simulink model "CoPT_TrqDesCoord1"  (R2016b)
settings: configuration reference "CodeGenConfigSet" (kept outside this file)
values from neighbouring files (symbols this model uses):
  DCS_OVRDS_ENGPRT = fi(1,State_int32)    [init_CoPT_TrqDesCoord.m]    (also in init_CoPT_TrqDesCoord_SIL.m)
  DCSOVRDSENGPRT_SY = fi(1,State_int32)    [init_CoPT_TrqDesCoord.m]    (also in init_CoPT_TrqDesCoord_SIL.m)
  DFFTLPRT_OVRDS_TSCINC = fi(1,State_int32)    [init_CoPT_TrqDesCoord.m]    (also in init_CoPT_TrqDesCoord_SIL.m)
  DFFTLPRTOVRDSTSCINC_SY = fi(1,State_int32)    [init_CoPT_TrqDesCoord.m]    (also in init_CoPT_TrqDesCoord_SIL.m)
  PTPRT_OVRDS_SPDGOV = fi(1,State_int32)    [init_CoPT_TrqDesCoord.m]    (also in init_CoPT_TrqDesCoord_SIL.m)
  PTPRTOVRDSSPDGOV_SY = fi(0,State_int32)    [init_CoPT_TrqDesCoord.m]    (also in init_CoPT_TrqDesCoord_SIL.m)
libraries: simulink x6
settings Model: Creator=Wollf  LastModifiedBy=lenovo
settings ConfigSetRef: SourceLocation=Base Workspace

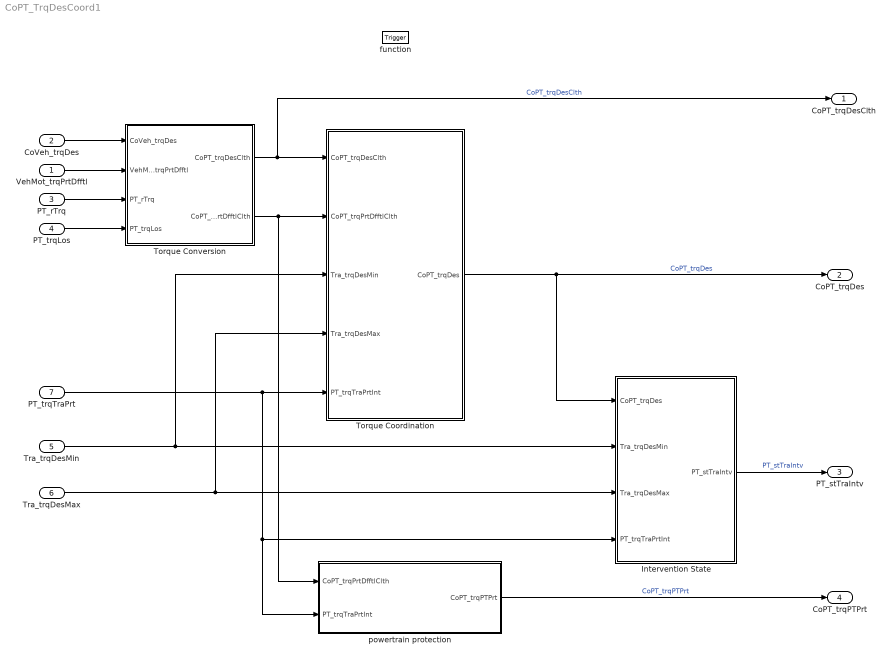
== system CoPT_TrqDesCoord1 ==
  VehMot_trqPrtDfftl : Inport  Tag=Nm  Description=Differential protection torque  OutMin=-3000  OutMax=3000  OutDataTypeStr=Trq_Nm
  CoVeh_trqDes : Inport  Tag=Nm  Description=Setpoint torque order to the drive train (gearbox output torque)  Port=2  OutMin=-3000  OutMax=3000  OutDataTypeStr=Trq_Nm
  PT_rTrq : Inport  Description=Powertrain torque ratio  Port=3  OutMin=-100  OutMax=100  OutDataTypeStr=TransRatio
  PT_trqLos : Inport  Tag=Nm  Description=Parameter for loss torque of the drive train  Port=4  OutMin=-3000  OutMax=3000  OutDataTypeStr=Trq_Nm
  Tra_trqDesMin : Inport  Tag=Nm  Description=Increment torque demand from gearbox  Port=5  OutMin=-3000  OutMax=3000  OutDataTypeStr=Trq_Nm
  Tra_trqDesMax : Inport  Tag=Nm  Description=Decrement torque demand from gearbox  Port=6  OutMin=-3000  OutMax=3000  OutDataTypeStr=Trq_Nm
  PT_trqTraPrt : Inport  Tag=Nm  Description=Maximum allowed inner torque  Port=7  OutMin=-3000  OutMax=3000  OutDataTypeStr=Trq_Nm
  function : TriggerPort  TriggerType=function-call  VariantControl=Variant
  Intervention State : Subsystem
  Torque Conversion : Subsystem
  Torque Coordination : Subsystem
  powertrain protection : Subsystem
  CoPT_trqDesClth : Outport  Tag=Nm  Description=Desired Clutch Torque  OutMin=-3000  OutMax=3000  OutDataTypeStr=Trq_Nm
  CoPT_trqDes : Outport  Tag=Nm  Description=Total torque order for torque actuator (clutch torque)  Port=2  OutMin=-3000  OutMax=3000  OutDataTypeStr=Trq_Nm
  PT_stTraIntv : Outport  Description=Status of torque access gearbox interventions  Port=3  OutMin=0  OutMax=255  OutDataTypeStr=State_uint8
  CoPT_trqPTPrt : Outport  Tag=Nm  Description=Drive train protection torque (clutch torque)  Port=4  OutMin=-3000  OutMax=3000  OutDataTypeStr=Trq_Nm
  wires:
  VehMot_trqPrtDfftl/1 -> Torque Conversion/2(VehMot_trqPrtDfftl)
  PT_rTrq/1 -> Torque Conversion/3(PT_rTrq)
  PT_trqLos/1 -> Torque Conversion/4(PT_trqLos)
  PT_trqTraPrt/1 -> powertrain protection/2(PT_trqTraPrtInt), Intervention State/4(PT_trqTraPrtInt), Torque Coordination/5(PT_trqTraPrtInt)
  Intervention State/1(PT_stTraIntv) -> PT_stTraIntv/1  "PT_stTraIntv"
  Torque Conversion/1(CoPT_trqDesClth) -> CoPT_trqDesClth/1, Torque Coordination/1(CoPT_trqDesClth)  "CoPT_trqDesClth"
  Torque Coordination/1(CoPT_trqDes) -> CoPT_trqDes/1, Intervention State/1(CoPT_trqDes)  "CoPT_trqDes"
  Torque Conversion/2(CoPT_trqPrtDfftlClth) -> powertrain protection/1(CoPT_trqPrtDfftlClth), Torque Coordination/2(CoPT_trqPrtDfftlClth)
  powertrain protection/1(CoPT_trqPTPrt) -> CoPT_trqPTPrt/1  "CoPT_trqPTPrt"
  CoVeh_trqDes/1 -> Torque Conversion/1(CoVeh_trqDes)
  Tra_trqDesMax/1 -> Intervention State/3(Tra_trqDesMax), Torque Coordination/4(Tra_trqDesMax)
  Tra_trqDesMin/1 -> Intervention State/2(Tra_trqDesMin), Torque Coordination/3(Tra_trqDesMin)

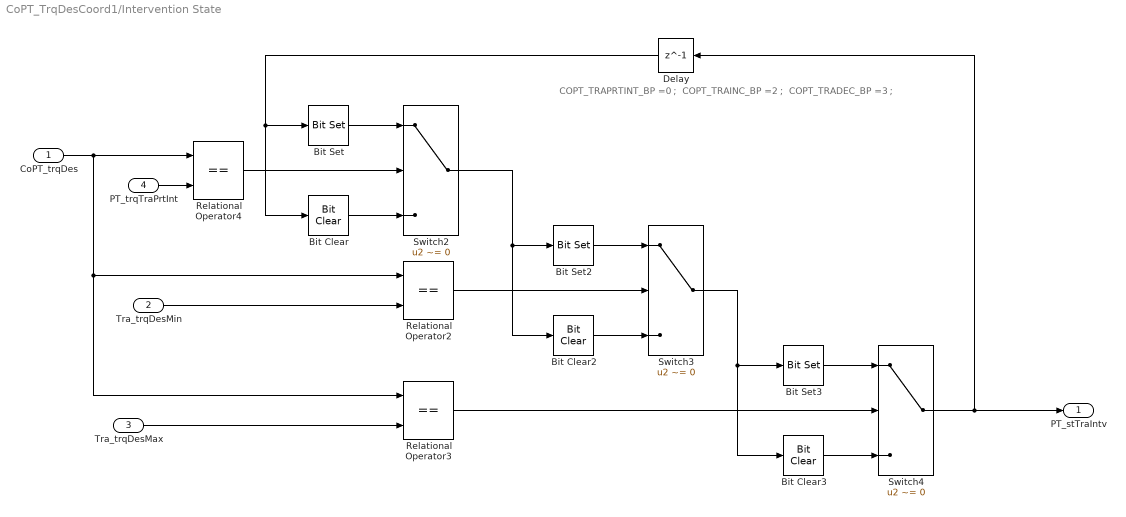
== system CoPT_TrqDesCoord1/Intervention State ==
  note: COPT_TRAPRTINT_BP =0；
      |
      | COPT_TRAINC_BP =2；
      | COPT_TRADEC_BP =3；
  CoPT_trqDes : Inport
  Tra_trqDesMin : Inport  Port=2
  Tra_trqDesMax : Inport  Port=3
  PT_trqTraPrtInt : Inport  Port=4
  Bit Clear : simulink/Logic and Bit Operations/Bit Clear  iBit=0
  Bit Clear2 : simulink/Logic and Bit Operations/Bit Clear  iBit=2
  Bit Clear3 : simulink/Logic and Bit Operations/Bit Clear  iBit=3
  Bit Set : simulink/Logic and Bit Operations/Bit Set  iBit=0
  Bit Set2 : simulink/Logic and Bit Operations/Bit Set  iBit=2
  Bit Set3 : simulink/Logic and Bit Operations/Bit Set  iBit=3
  Delay : Delay  DelayLength=1  InitialCondition=0
  Relational Operator2 : RelationalOperator  Operator===  OutDataTypeStr=boolean  RndMeth=Simplest  InputSameDT=on
  Relational Operator3 : RelationalOperator  Operator===  OutDataTypeStr=boolean  RndMeth=Simplest  InputSameDT=on
  Relational Operator4 : RelationalOperator  Operator===  OutDataTypeStr=boolean  RndMeth=Simplest  InputSameDT=on
  Switch2 : Switch  Criteria=u2 ~= 0  InputSameDT=on
  Switch3 : Switch  Criteria=u2 ~= 0  InputSameDT=on
  Switch4 : Switch  Criteria=u2 ~= 0  InputSameDT=on
  PT_stTraIntv : Outport
  wires:
  Bit Clear/1 -> Switch2/3
  CoPT_trqDes/1 -> Relational Operator4/1, Relational Operator2/1, Relational Operator3/1
  PT_trqTraPrtInt/1 -> Relational Operator4/2
  Tra_trqDesMin/1 -> Relational Operator2/2
  Bit Set/1 -> Switch2/1
  Relational Operator4/1 -> Switch2/2
  Bit Set3/1 -> Switch4/1
  Bit Clear3/1 -> Switch4/3
  Switch3/1 -> Bit Clear3/1, Bit Set3/1
  Relational Operator3/1 -> Switch4/2
  Switch2/1 -> Bit Clear2/1, Bit Set2/1
  Bit Clear2/1 -> Switch3/3
  Bit Set2/1 -> Switch3/1
  Relational Operator2/1 -> Switch3/2
  Tra_trqDesMax/1 -> Relational Operator3/2
  Switch4/1 -> PT_stTraIntv/1, Delay/1
  Delay/1 -> Bit Set/1, Bit Clear/1

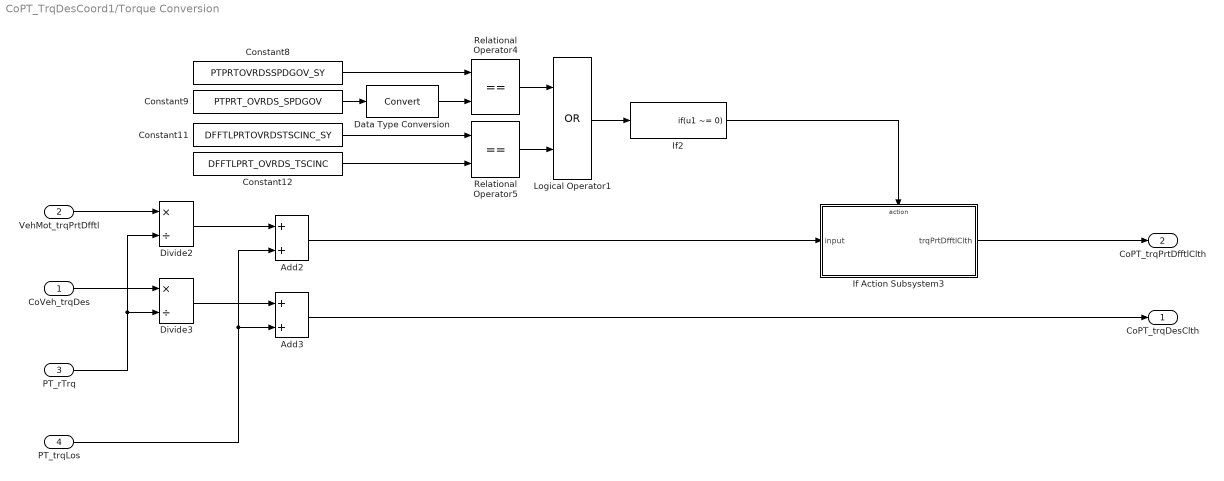
== system CoPT_TrqDesCoord1/Torque Conversion ==
  CoVeh_trqDes : Inport
  VehMot_trqPrtDfftl : Inport  Port=2
  PT_rTrq : Inport  Port=3
  PT_trqLos : Inport  Port=4
  Add2 : Sum  InputSameDT=on
  Add3 : Sum  InputSameDT=on
  Constant11 : Constant  Value=DFFTLPRTOVRDSTSCINC_SY
  Constant12 : Constant  Value=DFFTLPRT_OVRDS_TSCINC
  Constant8 : Constant  Value=PTPRTOVRDSSPDGOV_SY
  Constant9 : Constant  Value=PTPRT_OVRDS_SPDGOV
  Data Type Conversion : DataTypeConversion
  Divide2 : Product  Inputs=*/  OutDataTypeStr=Trq_Nm
  Divide3 : Product  Inputs=*/  OutDataTypeStr=Trq_Nm
  If Action Subsystem3 : Subsystem  TreatAsAtomicUnit=on
  If2 : If  IfExpression=u1 ~= 0  ShowElse=off
  Logical Operator1 : Logic  Operator=OR  OutDataTypeStr=boolean
  Relational Operator4 : RelationalOperator  Operator===  OutDataTypeStr=boolean  RndMeth=Simplest  InputSameDT=on
  Relational Operator5 : RelationalOperator  Operator===  OutDataTypeStr=boolean  RndMeth=Simplest  InputSameDT=on
  CoPT_trqDesClth : Outport
  CoPT_trqPrtDfftlClth : Outport  Port=2
  wires:
  Data Type Conversion/1 -> Relational Operator4/2
  CoVeh_trqDes/1 -> Divide3/1
  Divide3/1 -> Add3/1
  Divide2/1 -> Add2/1
  Relational Operator4/1 -> Logical Operator1/1
  Relational Operator5/1 -> Logical Operator1/2
  PT_rTrq/1 -> Divide3/2, Divide2/2
  VehMot_trqPrtDfftl/1 -> Divide2/1
  Constant11/1 -> Relational Operator5/1
  PT_trqLos/1 -> Add3/2, Add2/2
  If2/1 -> If Action Subsystem3/Action
  Logical Operator1/1 -> If2/1
  If Action Subsystem3/1(trqPrtDfftlClth) -> CoPT_trqPrtDfftlClth/1
  Add2/1 -> If Action Subsystem3/1(input)
  Constant8/1 -> Relational Operator4/1
  Constant9/1 -> Data Type Conversion/1
  Constant12/1 -> Relational Operator5/2
  Add3/1 -> CoPT_trqDesClth/1

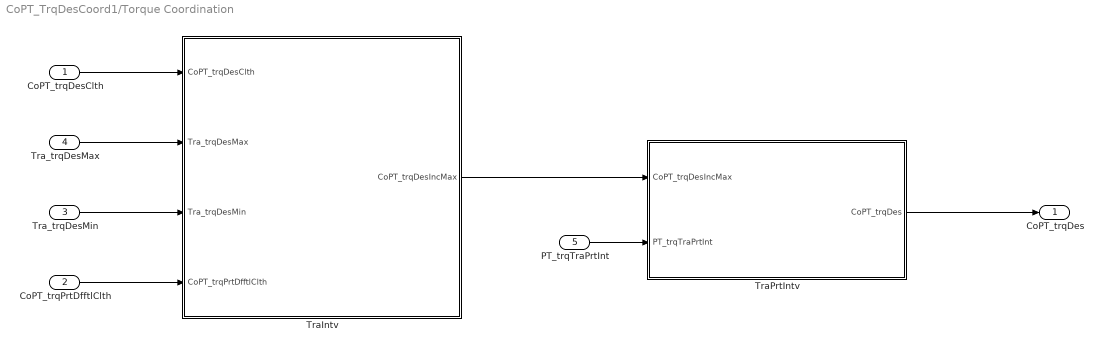
== system CoPT_TrqDesCoord1/Torque Coordination ==
  CoPT_trqDesClth : Inport
  CoPT_trqPrtDfftlClth : Inport  Port=2
  Tra_trqDesMin : Inport  Port=3
  Tra_trqDesMax : Inport  Port=4
  PT_trqTraPrtInt : Inport  Port=5
  TraIntv : Subsystem
  TraPrtIntv : Subsystem
  CoPT_trqDes : Outport
  wires:
  PT_trqTraPrtInt/1 -> TraPrtIntv/2(PT_trqTraPrtInt)
  TraPrtIntv/1(CoPT_trqDes) -> CoPT_trqDes/1
  CoPT_trqDesClth/1 -> TraIntv/1(CoPT_trqDesClth)
  Tra_trqDesMax/1 -> TraIntv/2(Tra_trqDesMax)
  Tra_trqDesMin/1 -> TraIntv/3(Tra_trqDesMin)
  CoPT_trqPrtDfftlClth/1 -> TraIntv/4(CoPT_trqPrtDfftlClth)
  TraIntv/1(CoPT_trqDesIncMax) -> TraPrtIntv/1(CoPT_trqDesIncMax)

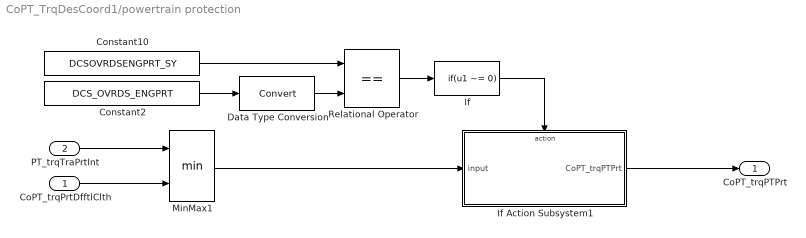
== system CoPT_TrqDesCoord1/powertrain protection ==
  CoPT_trqPrtDfftlClth : Inport
  PT_trqTraPrtInt : Inport  Port=2
  Constant10 : Constant  Value=DCSOVRDSENGPRT_SY
  Constant2 : Constant  Value=DCS_OVRDS_ENGPRT
  Data Type Conversion : DataTypeConversion
  If : If  IfExpression=u1 ~= 0  ShowElse=off
  If Action Subsystem1 : Subsystem  TreatAsAtomicUnit=on
  MinMax1 : MinMax  Inputs=2  InputSameDT=on
  Relational Operator : RelationalOperator  Operator===  OutDataTypeStr=boolean  RndMeth=Simplest  InputSameDT=on
  CoPT_trqPTPrt : Outport
  wires:
  PT_trqTraPrtInt/1 -> MinMax1/1
  CoPT_trqPrtDfftlClth/1 -> MinMax1/2
  If/1 -> If Action Subsystem1/Action
  MinMax1/1 -> If Action Subsystem1/1(input)
  Relational Operator/1 -> If/1
  Constant2/1 -> Data Type Conversion/1
  Constant10/1 -> Relational Operator/1
  If Action Subsystem1/1(CoPT_trqPTPrt) -> CoPT_trqPTPrt/1
  Data Type Conversion/1 -> Relational Operator/2

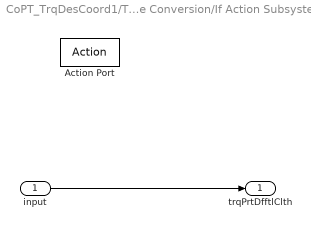
== system CoPT_TrqDesCoord1/Torque Conversion/If Action Subsystem3 ==
  input : Inport
  Action Port : ActionPort  ActionType=then
  trqPrtDfftlClth : Outport
  wires:
  input/1 -> trqPrtDfftlClth/1

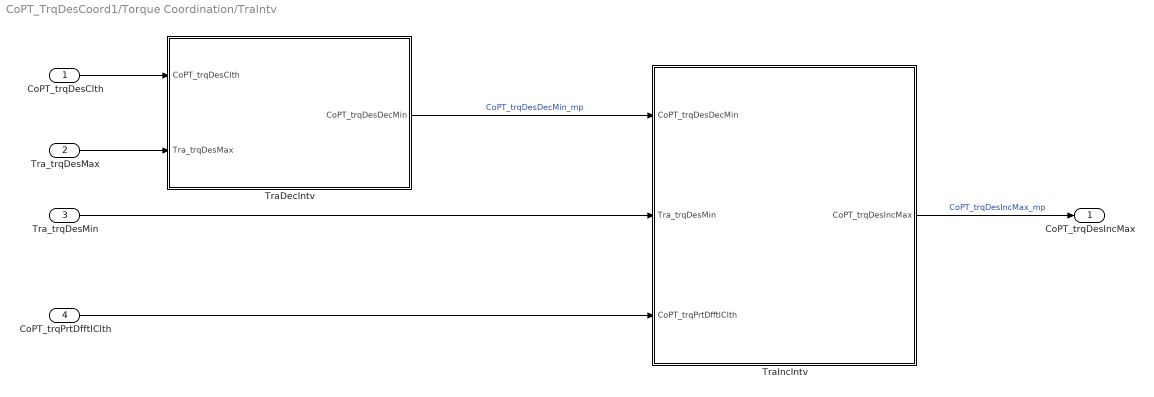
== system CoPT_TrqDesCoord1/Torque Coordination/TraIntv ==
  CoPT_trqDesClth : Inport
  Tra_trqDesMax : Inport  Port=2
  Tra_trqDesMin : Inport  Port=3
  CoPT_trqPrtDfftlClth : Inport  Port=4
  TraDecIntv : Subsystem
  TraIncIntv : Subsystem
  CoPT_trqDesIncMax : Outport
  wires:
  Tra_trqDesMin/1 -> TraIncIntv/2(Tra_trqDesMin)
  TraIncIntv/1(CoPT_trqDesIncMax) -> CoPT_trqDesIncMax/1  "CoPT_trqDesIncMax_mp"
  CoPT_trqPrtDfftlClth/1 -> TraIncIntv/3(CoPT_trqPrtDfftlClth)
  Tra_trqDesMax/1 -> TraDecIntv/2(Tra_trqDesMax)
  CoPT_trqDesClth/1 -> TraDecIntv/1(CoPT_trqDesClth)
  TraDecIntv/1(CoPT_trqDesDecMin) -> TraIncIntv/1(CoPT_trqDesDecMin)  "CoPT_trqDesDecMin_mp"

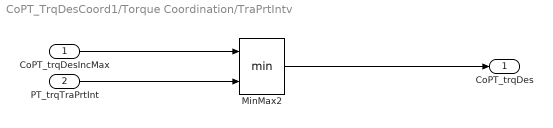
== system CoPT_TrqDesCoord1/Torque Coordination/TraPrtIntv ==
  CoPT_trqDesIncMax : Inport
  PT_trqTraPrtInt : Inport  Port=2
  MinMax2 : MinMax  Inputs=2  InputSameDT=on
  CoPT_trqDes : Outport
  wires:
  MinMax2/1 -> CoPT_trqDes/1
  CoPT_trqDesIncMax/1 -> MinMax2/1
  PT_trqTraPrtInt/1 -> MinMax2/2

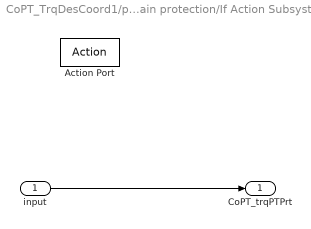
== system CoPT_TrqDesCoord1/powertrain protection/If Action Subsystem1 ==
  input : Inport
  Action Port : ActionPort  ActionType=then
  CoPT_trqPTPrt : Outport
  wires:
  input/1 -> CoPT_trqPTPrt/1

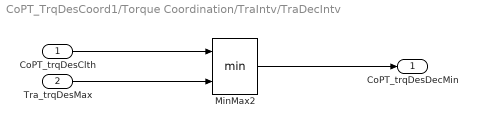
== system CoPT_TrqDesCoord1/Torque Coordination/TraIntv/TraDecIntv ==
  CoPT_trqDesClth : Inport
  Tra_trqDesMax : Inport  Port=2
  MinMax2 : MinMax  Inputs=2  InputSameDT=on
  CoPT_trqDesDecMin : Outport
  wires:
  MinMax2/1 -> CoPT_trqDesDecMin/1
  CoPT_trqDesClth/1 -> MinMax2/1
  Tra_trqDesMax/1 -> MinMax2/2

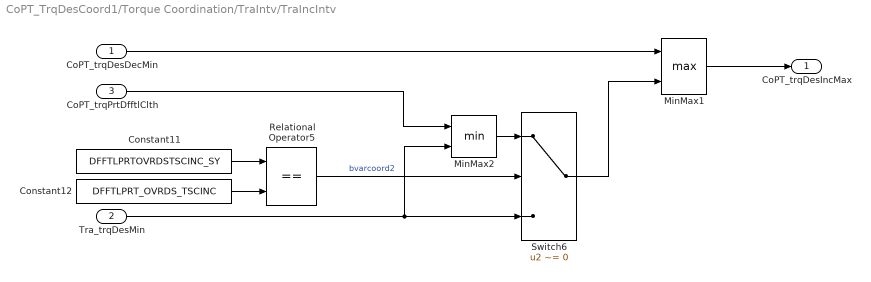
== system CoPT_TrqDesCoord1/Torque Coordination/TraIntv/TraIncIntv ==
  CoPT_trqDesDecMin : Inport
  Tra_trqDesMin : Inport  Port=2
  CoPT_trqPrtDfftlClth : Inport  Port=3
  Constant11 : Constant  Value=DFFTLPRTOVRDSTSCINC_SY
  Constant12 : Constant  Value=DFFTLPRT_OVRDS_TSCINC
  MinMax1 : MinMax  Function=max  Inputs=2  InputSameDT=on
  MinMax2 : MinMax  Inputs=2  InputSameDT=on
  Relational Operator5 : RelationalOperator  Operator===  OutDataTypeStr=boolean  RndMeth=Simplest  InputSameDT=on
  Switch6 : Switch  Criteria=u2 ~= 0  InputSameDT=on
  CoPT_trqDesIncMax : Outport
  wires:
  MinMax1/1 -> CoPT_trqDesIncMax/1
  Constant12/1 -> Relational Operator5/2
  Constant11/1 -> Relational Operator5/1
  CoPT_trqPrtDfftlClth/1 -> MinMax2/1
  CoPT_trqDesDecMin/1 -> MinMax1/1
  Relational Operator5/1 -> Switch6/2  "bvarcoord2"
  Tra_trqDesMin/1 -> MinMax2/2, Switch6/3
  MinMax2/1 -> Switch6/1
  Switch6/1 -> MinMax1/2
